simulink library "Flow_Mixer_basic"  (Simulink 8.2)
settings: Solver=ode45  StartTime=0.0  StopTime=10.0  RelTol=1e-3
undefined symbols (not defined in the file): DiameterLastPiece, DPConstant, DPLinear, DPQuadratic, FluidMix, FluidType, ID, MassFlow, Pressure, Temperature
libraries: carnot x1
settings Model: Creator=lena.frank  LastModifiedBy=drhf

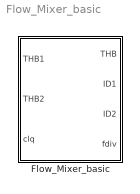
== system Flow_Mixer_basic ==
  Flow_Mixer_basic : Subsystem  mask(Flow Mixer Basic){}
      mask help:
      | The flow mixer calculated the temperature and massflow of 2 entering flows.
      | The temperature is calculated in the block Mix_T_Mdot.
      | The flow diversion fdiv (feed back to the flow diverter) takes care that the pressure drop in the 2 branches is the same. The resulting pressure drop coefficients are calulated in the s-function mix_flow (uses solve_quadratic_equation in Carlib).
      mask Help: web(fullfile(path_carnot('help'),'Flow_Mixer_basic.html'),'-helpbrowser')
      mask Display: disp('Flow\nMixer')

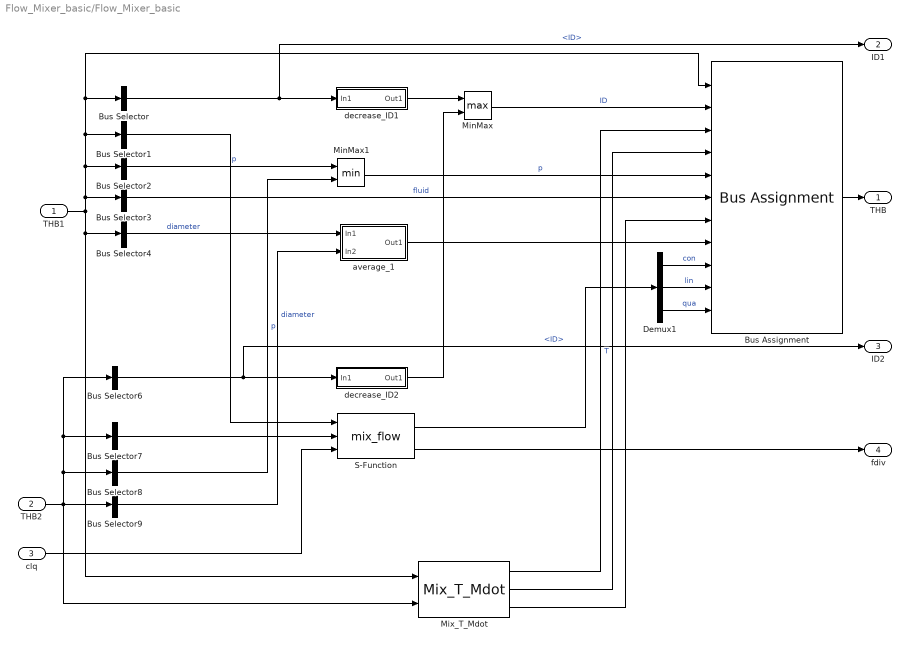
== system Flow_Mixer_basic/Flow_Mixer_basic ==
  THB1 : Inport
  THB2 : Inport  Port=2
  clq : Inport  Port=3
  Bus Assignment : BusAssignment  AssignedSignals=ID,Temperature,MassFlow,Pressure,FluidType,FluidMix,DiameterLastPiece,DPConstant,DPLinear,DPQuadratic
  Bus Selector : BusSelector  OutputSignals=ID
  Bus Selector1 : BusSelector  OutputSignals=ID,DPConstant,DPLinear,DPQuadratic  OutputAsBus=on
  Bus Selector2 : BusSelector  OutputSignals=Pressure  OutputAsBus=on
  Bus Selector3 : BusSelector  OutputSignals=FluidType  OutputAsBus=on
  Bus Selector4 : BusSelector  OutputSignals=DiameterLastPiece  OutputAsBus=on
  Bus Selector6 : BusSelector  OutputSignals=ID
  Bus Selector7 : BusSelector  OutputSignals=ID,DPConstant,DPLinear,DPQuadratic  OutputAsBus=on
  Bus Selector8 : BusSelector  OutputSignals=Pressure  OutputAsBus=on
  Bus Selector9 : BusSelector  OutputSignals=DiameterLastPiece  OutputAsBus=on
  Demux1 : Demux  Outputs=3
  MinMax : MinMax  Function=max  Inputs=2
  MinMax1 : MinMax  Inputs=2
  Mix_T_Mdot : carnot/Basic/Hydraulics/Mix_T_Mdot  mixcalc=Tmix = (mdot1*T1 + mdot2*T2)/(mdot1+mdot2)
  S-Function : S-Function  FunctionName=mix_flow  EnableBusSupport=off
  average_1 : Subsystem
  decrease_ID1 : Subsystem
  decrease_ID2 : Subsystem
  THB : Outport
  ID1 : Outport  Port=2
  ID2 : Outport  Port=3
  fdiv : Outport  Port=4
  wires:
  THB1/1 -> Bus Selector1/1, Bus Selector/1, Bus Assignment/1, Bus Selector2/1, Bus Selector3/1, Mix_T_Mdot/1, Bus Selector4/1
  Bus Selector/1 -> decrease_ID1/1(In1), ID1/1  "<ID>"
  decrease_ID1/1(Out1) -> MinMax/1
  decrease_ID2/1(Out1) -> MinMax/2
  MinMax/1 -> Bus Assignment/2  "ID"
  Bus Selector3/1 -> Bus Assignment/6  "fluid"
  THB2/1 -> Mix_T_Mdot/2, Bus Selector7/1, Bus Selector6/1, Bus Selector8/1, Bus Selector9/1
  Bus Selector6/1 -> decrease_ID2/1(In1), ID2/1  "<ID>"
  Bus Selector8/1 -> MinMax1/2  "p"
  Bus Selector4/1 -> average_1/1(In1)  "diameter"
  Bus Selector9/1 -> average_1/2(In2)  "diameter"
  average_1/1(Out1) -> Bus Assignment/8
  MinMax1/1 -> Bus Assignment/5  "p"
  Bus Selector1/1 -> S-Function/1
  Demux1/1 -> Bus Assignment/9  "con"
  Demux1/2 -> Bus Assignment/10  "lin"
  Demux1/3 -> Bus Assignment/11  "qua"
  S-Function/1 -> Demux1/1
  Mix_T_Mdot/1 -> Bus Assignment/3  "T"
  Mix_T_Mdot/3 -> Bus Assignment/7
  Mix_T_Mdot/2 -> Bus Assignment/4
  Bus Selector2/1 -> MinMax1/1  "p"
  Bus Selector7/1 -> S-Function/2
  Bus Assignment/1 -> THB/1
  clq/1 -> S-Function/3
  S-Function/2 -> fdiv/1

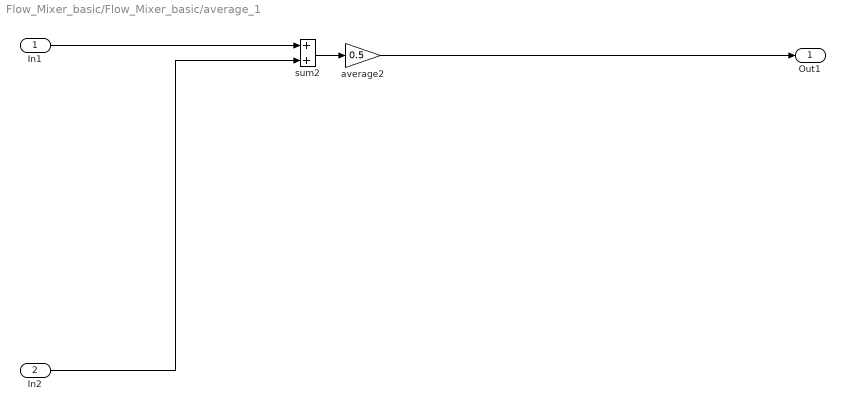
== system Flow_Mixer_basic/Flow_Mixer_basic/average_1 ==
  In1 : Inport
  In2 : Inport  Port=2
  average2 : Gain  Gain=0.5  SaturateOnIntegerOverflow=on  OutDataTypeStr=Inherit: Same as input  ParamDataTypeStr=Inherit: Same as input
  sum2 : Sum  SaturateOnIntegerOverflow=on  InputSameDT=on  OutDataTypeStr=Inherit: Same as first input
  Out1 : Outport
  wires:
  In2/1 -> sum2/2
  sum2/1 -> average2/1
  average2/1 -> Out1/1
  In1/1 -> sum2/1

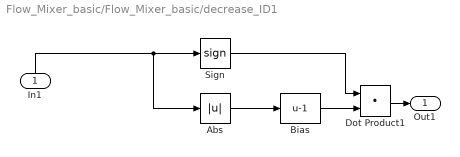
== system Flow_Mixer_basic/Flow_Mixer_basic/decrease_ID1 ==
  In1 : Inport
  Abs : Abs
  Bias : Bias  Bias=-1
  Dot Product1 : DotProduct  InputSameDT=on  OutDataTypeStr=Inherit: Inherit via internal rule
  Sign : Signum
  Out1 : Outport
  wires:
  In1/1 -> Abs/1, Sign/1
  Dot Product1/1 -> Out1/1
  Abs/1 -> Bias/1
  Sign/1 -> Dot Product1/1
  Bias/1 -> Dot Product1/2

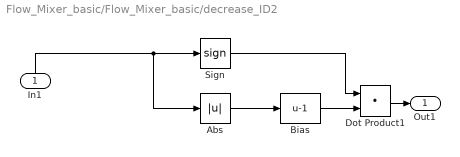
== system Flow_Mixer_basic/Flow_Mixer_basic/decrease_ID2 ==
  In1 : Inport
  Abs : Abs
  Bias : Bias  Bias=-1
  Dot Product1 : DotProduct  InputSameDT=on  OutDataTypeStr=Inherit: Inherit via internal rule
  Sign : Signum
  Out1 : Outport
  wires:
  Bias/1 -> Dot Product1/2
  Sign/1 -> Dot Product1/1
  Abs/1 -> Bias/1
  Dot Product1/1 -> Out1/1
  In1/1 -> Sign/1, Abs/1
